simulink model "ex"  (Simulink 7.1)
settings: Solver=ode5  StartTime=0.0  StopTime=10.0  RelTol=1e-3
settings Model: Creator=Administrator  LastModifiedBy=Administrator
settings DebuggingCC: SolverPrmCheckMsg=none
settings RTWCC: GenerateMakefile=off

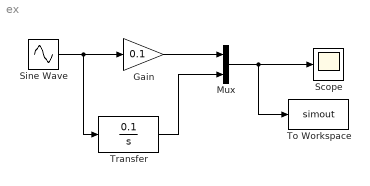
== system ex ==
  Gain : Gain  Gain=0.1  ParameterDataType=sfix(16)  ParameterScaling=2^0  OutDataType=sfix(16)  OutScaling=2^0
  Mux : Mux  Inputs=2
  Scope : Scope
  Sine Wave : Sin  SampleTime=0
  To Workspace : ToWorkspace  VariableName=simout  SampleTime=-1  SaveFormat=Array
  Transfer : TransferFcn  Numerator=0.1  Denominator=[1 0]
  wires:
  Sine Wave/1 -> Gain/1, Transfer/1
  Gain/1 -> Mux/1
  Mux/1 -> Scope/1, To Workspace/1
  Transfer/1 -> Mux/2
